simulink model "ROS_Android_Sensors"  (R2019b)
settings: Solver=FixedStepAuto  StartTime=0.0  StopTime=10.0  RelTol=1e-3
libraries: androidsensorlib x7, androidadvancedlib x2, simulink x1
settings Model: Creator=The MathWorks, Inc.  LastModifiedBy=Bilal
settings OptimizationCC: EnhancedBackFolding=on  PassReuseOutputArgsThreshold=0  MaxStackSize=64  OptimizeBlockOrder=speed  DifferentSizesBufferReuse=on  OptimizationCustomize=off
settings DebuggingCC: ParameterTunabilityLossMsg=error  ArithmeticOperatorsInVariantConditions=warning
settings HardwareCC: ProdBitPerPointer=32  ProdBitPerSizeT=32  ProdBitPerPtrDiffT=32  ProdLargestAtomicInteger=Long  ProdLargestAtomicFloat=Double  ProdWordSize=32  ProdHWDeviceType=ARM Compatible->ARM Cortex  UseEmbeddedCoderFeatures=off  UseSimulinkCoderFeatures=off
settings SFSimCC: MATLABDynamicMemAlloc=off  CustomCodeUndefinedFunction=UseInterfaceOnly
settings RTWCC: SystemTargetFile=ert.tlc  HardwareBoard=Android Device  TLCOptions="-aInlineSetEventsForThisBaseRateFcn=TLC_FALSE -aSuppressMultiTaskScheduler=TLC_FALSE  -aRateBasedStepFcn=0"  TemplateMakefile=ert_default_tmf  GenerateReport=on  RTWVerbose=off  Toolchain=Android SDK/NDK Tools  LaunchReport=on
settings CodeAppCC: ForceParamTrailComments=on  OperatorAnnotations=on
settings ERTTargetCC: ERTCustomFileBanners=off  SupportContinuousTime=on  SupportNonInlinedSFcns=on  RemoveResetFunc=off  ModelStepFunctionPrototypeControlCompliant=off

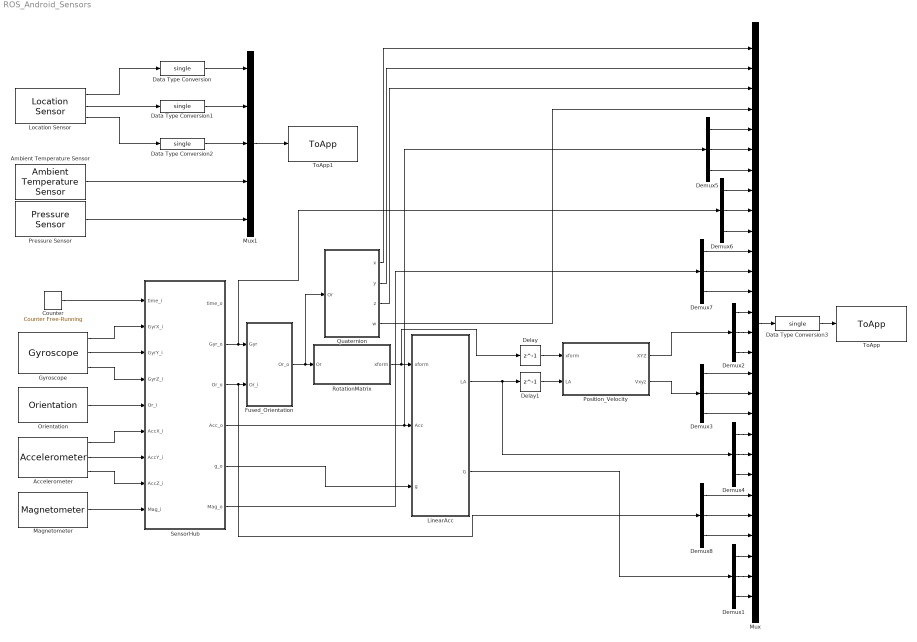
== system ROS_Android_Sensors ==
  Accelerometer : androidsensorlib/Accelerometer  OutputVector=off  SampleTime=0.01  BlockPlatform=Android
      settings: SourceProductName=Simulink Support Package for Android Devices  SourceProductBaseCode=ANDROID
  Ambient Temperature Sensor : androidsensorlib/Ambient Temperature Sensor  SampleTime=1  BlockPlatform=Android
      settings: SourceProductName=Simulink Support Package for Android Devices  SourceProductBaseCode=ANDROID
  Counter : simulink/Sources/Counter Free-Running  NumBits=16  tsamp=1
  Data Type Conversion{,1..3} (4 alike) : DataTypeConversion  OutDataTypeStr=single
  Delay : Delay  DelayLength=1  InitialCondition=0
  Delay1 : Delay  DelayLength=1  InitialCondition=0
  Demux{1..8} (8 alike) : Demux  Outputs=3
  Fused_Orientation : MATLAB Function  TreatAsAtomicUnit=on
  Gyroscope : androidsensorlib/Gyroscope  OutputVector=off  SampleTime=0.01  BlockPlatform=Android
      settings: SourceProductName=Simulink Support Package for Android Devices  SourceProductBaseCode=ANDROID
  LinearAcc : MATLAB Function  TreatAsAtomicUnit=on
  Location Sensor : androidsensorlib/Location Sensor  OutputVector=off  SampleTime=1  BlockPlatform=Android
      settings: SourceProductName=Simulink Support Package for Android Devices  SourceProductBaseCode=ANDROID
  Magnetometer : androidsensorlib/Magnetometer  SampleTime=0.01  SimulateUsing=Code generation
      settings: SourceProductName=Simulink Support Package for Android Devices  SourceProductBaseCode=ANDROID
  Mux : Mux  Inputs=28
  Mux1 : Mux  Inputs=5
  Orientation : androidsensorlib/Orientation  SampleTime=0.01  SimulateUsing=Code generation
      settings: SourceProductName=Simulink Support Package for Android Devices  SourceProductBaseCode=ANDROID
  Position_Velocity : MATLAB Function  TreatAsAtomicUnit=on
  Pressure Sensor : androidsensorlib/Pressure Sensor  SampleTime=1  BlockPlatform=Android
      settings: SourceProductName=Simulink Support Package for Android Devices  SourceProductBaseCode=ANDROID
  Quaternion : MATLAB Function  TreatAsAtomicUnit=on
  RotationMatrix : MATLAB Function  TreatAsAtomicUnit=on
  SensorHub : MATLAB Function  TreatAsAtomicUnit=on
  ToApp : androidadvancedlib/ToApp  FunctionName=ROSPublishFast  NumInputs=1
      settings: SourceProductName=Simulink Support Package for Android Devices  SourceProductBaseCode=ANDROID
  ToApp1 : androidadvancedlib/ToApp  FunctionName=ROSPublishSlow  NumInputs=1
      settings: SourceProductName=Simulink Support Package for Android Devices  SourceProductBaseCode=ANDROID
  wires:
  LinearAcc/1(LA) -> Demux4/1, Delay1/1
  Delay1/1 -> Position_Velocity/2(LA)
  Demux6/3 -> Mux/10
  Delay/1 -> Position_Velocity/1(xform)
  RotationMatrix/1(xform) -> Delay/1, LinearAcc/1(xform)
  Demux5/3 -> Mux/7
  Demux2/2 -> Mux/15
  Demux2/1 -> Mux/14
  SensorHub/3(Or_o) -> Demux8/1, Fused_Orientation/2(Or_i)
  Fused_Orientation/1(Or_o) -> Quaternion/1(Or), RotationMatrix/1(Or)
  Mux/1 -> Data Type Conversion3/1
  SensorHub/4(Acc_o) -> Demux5/1, LinearAcc/2(Acc)
  Accelerometer/1 -> SensorHub/6(AccX_i)
  Magnetometer/1 -> SensorHub/9(Mag_i)
  Accelerometer/3 -> SensorHub/8(AccZ_i)
  Accelerometer/2 -> SensorHub/7(AccY_i)
  Gyroscope/1 -> SensorHub/2(GyrX_i)
  Counter/1 -> SensorHub/1(time_i)
  Gyroscope/3 -> SensorHub/4(GyrZ_i)
  Location Sensor/3 -> Data Type Conversion2/1
  Gyroscope/2 -> SensorHub/3(GyrY_i)
  Pressure Sensor/1 -> Mux1/5
  Location Sensor/2 -> Data Type Conversion1/1
  Data Type Conversion/1 -> Mux1/1
  Data Type Conversion1/1 -> Mux1/2
  Demux6/1 -> Mux/8
  Position_Velocity/2(Vxyz) -> Demux3/1
  Demux5/1 -> Mux/5
  Location Sensor/1 -> Data Type Conversion/1
  SensorHub/2(Gyr_o) -> Demux6/1, Fused_Orientation/1(Gyr)
  Demux8/1 -> Mux/23
  SensorHub/6(Mag_o) -> Demux7/1
  Demux6/2 -> Mux/9
  Data Type Conversion2/1 -> Mux1/3
  Demux5/2 -> Mux/6
  Orientation/1 -> SensorHub/5(Or_i)
  Demux8/3 -> Mux/25
  Demux7/1 -> Mux/11
  Demux7/3 -> Mux/13
  Demux8/2 -> Mux/24
  Quaternion/2(y) -> Mux/2
  Demux2/3 -> Mux/16
  Mux1/1 -> ToApp1/1
  Demux4/2 -> Mux/21
  Quaternion/4(w) -> Mux/4
  Demux3/3 -> Mux/19
  Quaternion/3(z) -> Mux/3
  Quaternion/1(x) -> Mux/1
  Demux3/2 -> Mux/18
  Demux4/1 -> Mux/20
  Demux3/1 -> Mux/17
  Demux4/3 -> Mux/22
  Demux7/2 -> Mux/12
  Ambient Temperature Sensor/1 -> Mux1/4
  SensorHub/5(g_o) -> LinearAcc/3(g)
  Position_Velocity/1(XYZ) -> Demux2/1
  Demux1/1 -> Mux/26
  Demux1/2 -> Mux/27
  Demux1/3 -> Mux/28
  LinearAcc/2(G) -> Demux1/1
  Data Type Conversion3/1 -> ToApp/1

== matlab function ROS_Android_Sensors/LinearAcc ==
  data: xform input; LA output; Acc input; g input; G output
function [LA,G] = removeG(xform,Acc,g)
    G = xform'*[0;0;g];
    LA = (Acc-G);
%     Best way to debug this module is to visualize on a scope

== matlab function ROS_Android_Sensors/RotationMatrix ==
  data: Or input; xform output
function xform = rot_mat(Or)
roll = double(Or(1));
pitch = double(Or(2));
yaw = double(Or(3));

rz = [cos(yaw) -sin(yaw) 0;sin(yaw) cos(yaw) 0;0 0 1];
ry = [cos(pitch) 0 sin(pitch);0 1 0;-sin(pitch) 0 cos(pitch)];
rx = [1 0 0;0 cos(roll) -sin(roll);0 sin(roll) cos(roll)];
xform = (rz*ry*rx);    %Rotation Matrix

== matlab function ROS_Android_Sensors/Position_Velocity ==
  data: xform input; LA input; XYZ output; Vxyz output
function [XYZ,Vxyz] = XYZ_UVW(xform,LA)
persistent xyz; %Position
persistent uvw; %Velocity
    if(isempty(xyz))
        xyz = double([0;0;0]);
        uvw = double([0;0;0]);
    end

% xform = eye(3); %enable for testing only
% LA = [0;0;0];
% LA(1) = 0.1;

XYZ = xyz + (xform*uvw*0.01);  %Update position vector using previous velocity vector
xyz = XYZ;

Vxyz = uvw + LA*0.01;   %Update velocity vector
uvw = Vxyz;

== matlab function ROS_Android_Sensors/SensorHub ==
  data: time_i input; time_o output; Gyr_o output; GyrX_i input; GyrY_i input; GyrZ_i input; Or_i input; AccX_i input; AccY_i input; AccZ_i input; Mag_i input; Or_o output; Acc_o output; g_o output; Mag_o output
function  [time_o,Gyr_o,Or_o,Acc_o,g_o,Mag_o] = SensorConditioner(time_i,GyrX_i,GyrY_i,GyrZ_i,Or_i,AccX_i,AccY_i,AccZ_i,Mag_i)
% Axis transformation for Android->ROS framework
% Basic processing
% Type conversion

time_o = time_i;

% Smartphone axis are Z-Up, Y-Front, X-Right
%ROS axis are Z-Up, X-Front, Y-Left
AccX_o = double(AccY_i);
AccY_o = double(-AccX_i);
AccZ_o = double(AccZ_i);
Acc_o = [AccX_o;AccY_o;AccZ_o];

% Smartphone uses left-hand rule, ROS uses right-hand rule
GyrX_o = double(GyrY_i);
GyrY_o = double(-GyrX_i);
GyrZ_o = double(GyrZ_i);
Gyr_o = [GyrX_o;GyrY_o;GyrZ_o];

Mag_o = double(Mag_i)';

% IMPORTANT: Convert to radians "IF" Android project reads in Degrees!
Or_o = double([Or_i(2);Or_i(1);-Or_i(3)]);%*pi/180

if(time_i<10)
    Gyr_o = [0;0;0];
    Or_o = [0;0;0];
    Acc_o = [0;0;0];
    Mag_o = [0;0;0];
end

% Estimate 'g' by keeping phone stable during first 10 sec.
persistent g;
persistent n;
    if(isempty(g))
        g = double(9.8);
        n = 0;
    end
%     c = double(0.9);
    if(time_i<10)
%         g = sqrt(AccX_o^2+AccY_o^2+AccZ_o^2)*c + g*(1-c);
        g = g + sqrt(AccX_o^2+AccY_o^2+AccZ_o^2);
        n = n + 1;
        g_o = 0;
    else
        g_o = double(g/n);
    end

== matlab function ROS_Android_Sensors/Fused_Orientation ==
  data: Gyr input double; Or_i input; Or_o output double
function Or_o = fuse_Or(Gyr,Or_i)
persistent Or_p;
    if(isempty(Or_p))
        Or_p = double([0;0;0]);
    end
    
fuse_c = double(0.9); %[0 1] 0-Acc, 1-Gyro
dt = double(0.01);%Fixed delta-time

% Complementary Filter
Or_o = fuse_angles(Or_p + Gyr*dt,Or_i,fuse_c,1-fuse_c);
Or_p = Or_o;
end


function out = fuse_angles(a,b,aw,bw)
ca = cos(a);
cb = cos(b);
sa = sin(a);
sb = sin(b);
co = ca*aw+cb*bw;
so = sa*aw+sb*bw;
out = double(atan2(so,co));
end

== matlab function ROS_Android_Sensors/Quaternion ==
  data: Or input; x output; y output; z output; w output
function  [x,y,z,w] = eul2quat(Or)
roll = double(Or(1));
pitch = double(Or(2));
yaw = double(Or(3));

% Convert the quaternion to a yaw angle (zyx euler angle)
quat = eul2quat([yaw,roll,pitch]);
x = quat(1); y = quat(2); z = quat(3); w = quat(4);

end
